simulink model "Pendulo_No_Lineal"  (R2022b)
settings: Solver=VariableStepAuto  StartTime=0.0  StopTime=1.5  MaxStep=0.025  MinStep=0.02459  RelTol=1e-3
settings Model: Creator=Carlos Arturo  LastModifiedBy=Carlos Arturo

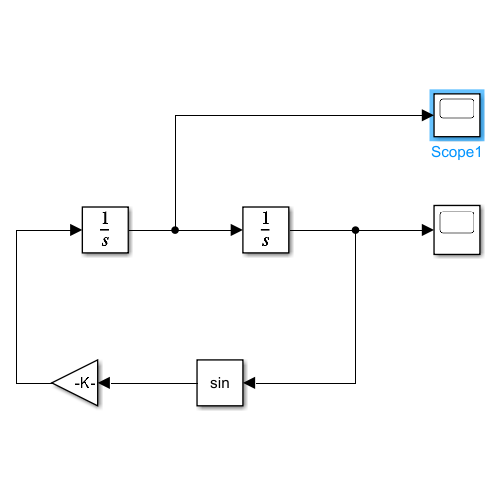
[thumbnail: Simulink's stored preview of the top-level diagram]
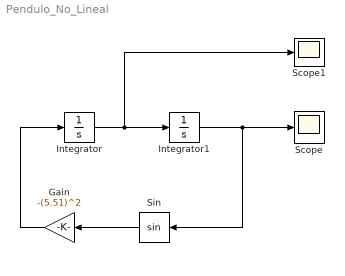
== system Pendulo_No_Lineal ==
  Gain : Gain  Gain=-(5.51)^2
  Integrator : Integrator
  Integrator1 : Integrator  InitialCondition=pi/18
  Scope : Scope
  Scope1 : Scope
  Sin : Trigonometry  ApproximationMethod=Lookup  NumberOfIterations=10  NumberOfDataPoints=100
  wires:
  Integrator/1 -> Scope1/1, Integrator1/1
  Integrator1/1 -> Sin/1, Scope/1
  Gain/1 -> Integrator/1
  Sin/1 -> Gain/1
